simulink model "exp1_p3"  (R2018a)
settings: Solver=VariableStepAuto  StartTime=0.0  StopTime=10.0  RelTol=1e-3
settings Model: Creator=asish  LastModifiedBy=asish

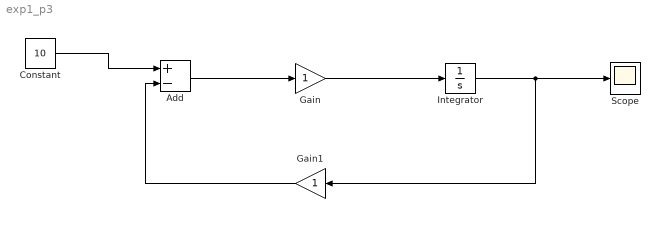
== system exp1_p3 ==
  Add : Sum  Inputs=+-
  Constant : Constant  Value=10
  Gain : Gain
  Gain1 : Gain
  Integrator : Integrator
  Scope : Scope
  wires:
  Gain/1 -> Integrator/1
  Add/1 -> Gain/1
  Integrator/1 -> Gain1/1, Scope/1
  Constant/1 -> Add/1
  Gain1/1 -> Add/2
